simulink model "CnvSet"  (R2018a)
settings: configuration reference "cs_ert" (kept outside this file)
settings Model: DataDictionary=CnvSet.sldd  Creator=zhoutinglin  LastModifiedBy=zhoutinglin

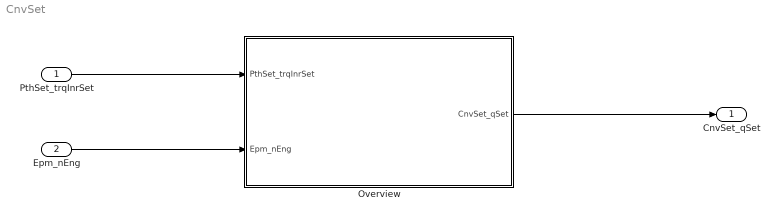
== system CnvSet ==
  PthSet_trqInrSet : Inport
  Epm_nEng : Inport  Port=2
  Overview : Subsystem
  CnvSet_qSet : Outport
  wires:
  PthSet_trqInrSet/1 -> Overview/1(PthSet_trqInrSet)
  Epm_nEng/1 -> Overview/2(Epm_nEng)
  Overview/1(CnvSet_qSet) -> CnvSet_qSet/1

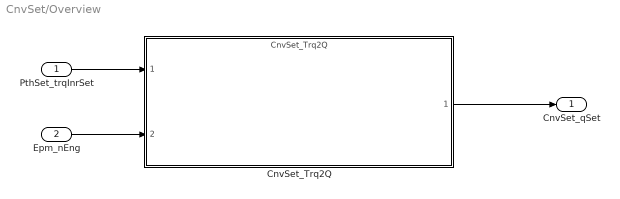
== system CnvSet/Overview ==
  PthSet_trqInrSet : Inport
  Epm_nEng : Inport  Port=2
  CnvSet_Trq2Q : ModelReference  ModelNameDialog=CnvSet_Trq2Q  SimulationMode=Normal  ModelReferenceVersion=1.63
  CnvSet_qSet : Outport
  wires:
  PthSet_trqInrSet/1 -> CnvSet_Trq2Q/1
  Epm_nEng/1 -> CnvSet_Trq2Q/2
  CnvSet_Trq2Q/1 -> CnvSet_qSet/1
